simulink model "aeroblk_hl20airframe"  (Simulink 6.0)
settings: Solver=ode45  StartTime=0.0  StopTime=1000.0  RelTol=1e-3
PreLoadFcn:
  | aeroblk_init_HL20
libraries: aeroblk_lib_HL20 x1
settings Model: Creator=The MathWorks Inc.  LastModifiedBy=batserve  ExtModeAutoUpdateStatusClock=off  BufferReuse=off
settings DataIOCC: SignalLoggingName=logsOut
settings OptimizationCC: BooleanDataType=off  OptimizeBlockIOStorage=off  BufferReuse=off  ExpressionFolding=off  LocalBlockOutputs=off
settings DebuggingCC: CheckExecutionContextPreStartOutputMsg=on  CheckExecutionContextRuntimeOutputMsg=on  SolverPrmCheckMsg=none
settings HardwareCC: TargetUnknown=on

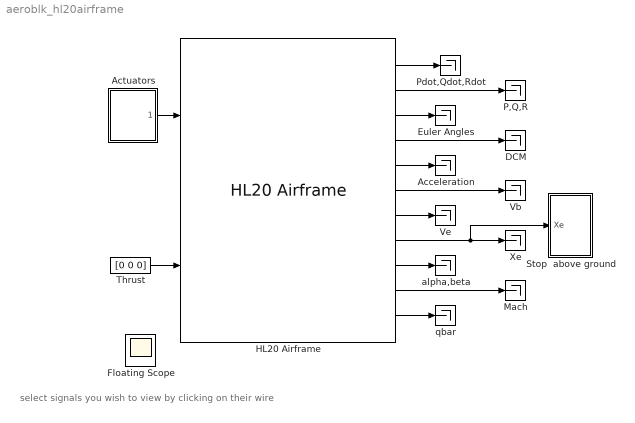
== system aeroblk_hl20airframe ==
  note: select signals you wish to view
      | by clicking on their wire
  Acceleration : Terminator
  Actuators : Subsystem  PropExecContextAcrossSSBoundary=on
  DCM : Terminator
  Euler Angles : Terminator
  Floating Scope : Scope
      settings: Floating=on  TimeRange=10  YMin=-7500  YMax=1000
  HL20 Airframe : aeroblk_lib_HL20/HL20 Airframe
  Mach : Terminator
  P,Q,R : Terminator
  Pdot,Qdot,Rdot : Terminator
  Stop  above ground : Subsystem  PropExecContextAcrossSSBoundary=on
  Thrust : Constant  Value=[0 0 0]
  Vb : Terminator
  Ve : Terminator
  Xe : Terminator
  alpha,beta : Terminator
  qbar : Terminator
  wires:
  Thrust/1 -> HL20 Airframe/2
  Actuators/1(Positions) -> HL20 Airframe/1
  HL20 Airframe/11 -> qbar/1
  HL20 Airframe/3 -> Euler Angles/1
  HL20 Airframe/5 -> Acceleration/1
  HL20 Airframe/6 -> Vb/1
  HL20 Airframe/1 -> Pdot,Qdot,Rdot/1
  HL20 Airframe/2 -> P,Q,R/1
  HL20 Airframe/7 -> Ve/1
  HL20 Airframe/8 -> Xe/1, Stop  above ground/1(Xe)
  HL20 Airframe/10 -> Mach/1
  HL20 Airframe/9 -> alpha,beta/1
  HL20 Airframe/4 -> DCM/1

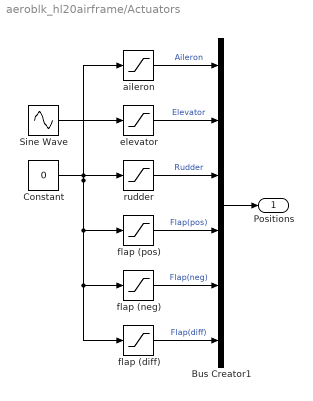
== system aeroblk_hl20airframe/Actuators ==
  Bus Creator1 : BusCreator  DialogController=Simulink.DDGSource_Bus  Inputs=6
  Constant : Constant  Value=0
  Sine Wave : Sin  Bias=10  SampleTime=0
  "aileron " : Saturate  UpperLimit=30  LowerLimit=-30
  elevator : Saturate  UpperLimit=30  LowerLimit=-30
  flap (diff) : Saturate  UpperLimit=60  LowerLimit=-60
  flap (neg) : Saturate  UpperLimit=0  LowerLimit=-60
  flap (pos) : Saturate  UpperLimit=60  LowerLimit=0
  rudder : Saturate  UpperLimit=60  LowerLimit=-60
  Positions : Outport
  wires:
  Bus Creator1/1 -> Positions/1
  flap (diff)/1 -> Bus Creator1/6  "Flap(diff)"
  flap (neg)/1 -> Bus Creator1/5  "Flap(neg)"
  rudder/1 -> Bus Creator1/3  "Rudder"
  elevator/1 -> Bus Creator1/2  "Elevator"
  "aileron "/1 -> Bus Creator1/1  "Aileron"
  flap (pos)/1 -> Bus Creator1/4  "Flap(pos)"
  Constant/1 -> rudder/1, flap (diff)/1, flap (neg)/1, flap (pos)/1, "aileron "/1
  Sine Wave/1 -> elevator/1

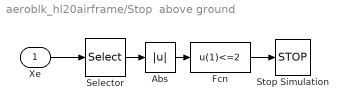
== system aeroblk_hl20airframe/Stop  above ground ==
  Xe : Inport  Port=1  LatchInput=off
  Abs : Abs  SaturateOnIntegerOverflow=on
  Fcn : Fcn  Expr=u(1)<=2
  Selector : Selector  Elements=3  InputPortWidth=3
  Stop Simulation : Stop
  wires:
  Selector/1 -> Abs/1
  Xe/1 -> Selector/1
  Abs/1 -> Fcn/1
  Fcn/1 -> Stop Simulation/1
